simulink model "PLL_Sim_Rev2"  (R2019b)
settings: Solver=VariableStepAuto  StartTime=0.0  StopTime=1  MaxStep=1000  MinStep=1e-10  RelTol=1e-2  AbsTol=1e-2
libraries: fl_lib x17, nesl_utility x8, ee_lib x6, impairlib x2
settings Model: Creator=connerhannon  LastModifiedBy=connerhannon
settings SolverCC: MaxConsecutiveZCs=10000000  MaxConsecutiveMinStep=1000000

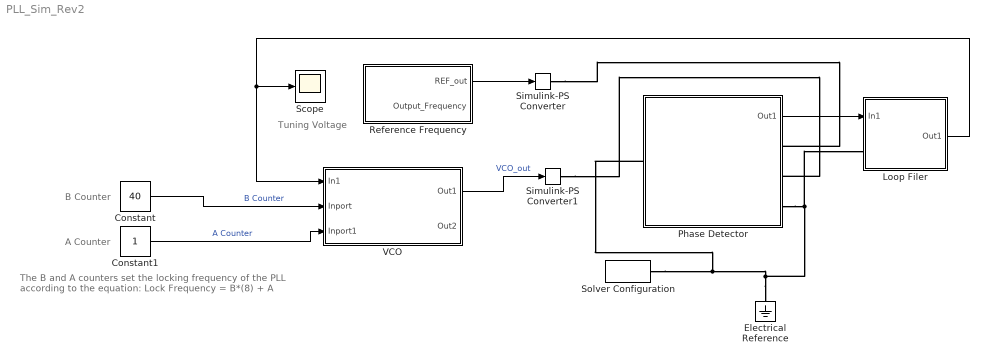
== system PLL_Sim_Rev2 ==
  note: Tuning Voltage
  note: B Counter
  note: The B and A counters set the locking frequency of the PLL
      | according to the equation:
      |
      | Lock Frequency = B*(8) + A
  note: A Counter
  Constant : Constant  Value=40
  Constant1 : Constant
  Electrical Reference : fl_lib/Electrical/Electrical Elements/Electrical Reference
  Loop Filer : Subsystem
  Phase Detector : Subsystem
  Reference Frequency : Subsystem
  Scope : Scope
  Simulink-PS Converter : nesl_utility/Simulink-PS Converter  PhysicalDomain=network_engine_domain  SubClassName=ps_input  LeftPortType=input  RightPortType=output  PseudoPeriodic=off  Frequencies=[]  NoiseDistribution=none  NoiseParameters=[]  Unit=1  AffineConversion=off  FilteringAndDerivatives=provide  SimscapeFilterOrder=1  InputFilterTimeConstant=0.001  UdotUserProvided=0
  Simulink-PS Converter1 : nesl_utility/Simulink-PS Converter  PhysicalDomain=network_engine_domain  SubClassName=ps_input  LeftPortType=input  RightPortType=output  PseudoPeriodic=off  Frequencies=[]  NoiseDistribution=none  NoiseParameters=[]  Unit=1  AffineConversion=off  FilteringAndDerivatives=provide  SimscapeFilterOrder=1  InputFilterTimeConstant=0.001  UdotUserProvided=0
  Solver Configuration : nesl_utility/Solver Configuration  PhysicalDomain=network_engine_domain  SubClassName=solver  LeftPortType=input  RightPortType=generic  Tones=[]  Harmonics=[]  SimulateNoise=off  Profile=off  UseLocalSampling=off  EnableSwitchedLinearOptims=on  FrequencyDomain=off  UseCCode=off  RelTol=0.001  AbsTol=1e-06  MinStep=1e-09  ToWorkspace=off  RevertToSquareIcSolve=off  NumHomotopyIterations=100  PhasorMode=off  PhasorModeNumHarmonics=1  DoDC=off  ResidualTolerance=1e-6  UseLocalSolver=off  LocalSolverChoice=NE_TRAPEZOIDAL_ADVANCER  LocalSolverSampleTime=1e-9  DoFixedCost=off  MaxNonlinIter=3  MaxModeIter=2  LinearAlgebra=auto  EquationFormulation=NE_TIME_EF  DelaysMemoryBudget=1024  AutomaticFiltering=on  FilteringTimeConstant=0.0001  PartitionStorageMethod=AS_NEEDED  PartitionMemoryBudget=1024  PartitionMethod=FAST
  VCO : Subsystem
  wires:
  Constant1/1 -> VCO/3(Inport1)  "A Counter"
  Reference Frequency/1(REF_out) -> Simulink-PS Converter/1
  Constant/1 -> VCO/2(Inport)  "B Counter"
  VCO/1(Out1) -> Simulink-PS Converter1/1  "VCO_out"
  Loop Filer/1(Out1) -> VCO/1(In1), Scope/1
  Phase Detector/1(Out1) -> Loop Filer/1(In1)
  connections:
  Electrical Reference/LConn1 -- Phase Detector/LConn1 -- Solver Configuration/RConn1 -- Phase Detector/RConn3 -- Loop Filer/LConn1
  Simulink-PS Converter/RConn1 -- Phase Detector/RConn1
  Simulink-PS Converter1/RConn1 -- Phase Detector/RConn2

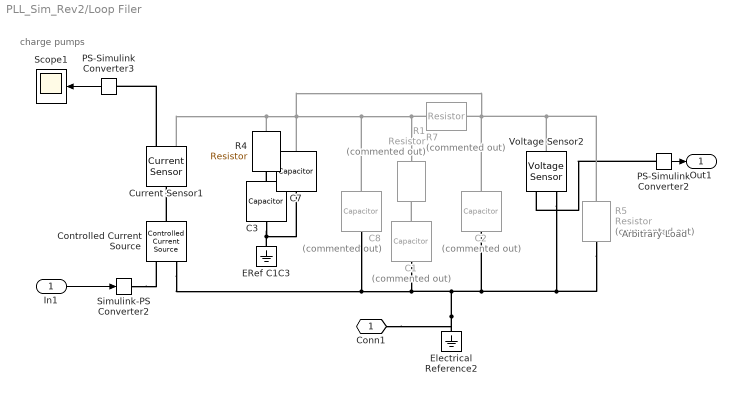
== system PLL_Sim_Rev2/Loop Filer ==
  note: Arbitrary Load
  note: charge pumps
  In1 : Inport
  C1 : fl_lib/Electrical/Electrical Elements/Capacitor  Commented=on  c=80 nF  r=1e-6 Ohm  g=0 1/Ohm  i_specify=off  i_priority=High  i=0 A  i_nominal_specify=off  i_nominal_unit=A  i_nominal_value=1  v_specify=off  v_priority=High  v=0 V  v_nominal_specify=off  v_nominal_unit=V  v_nominal_value=1  vc_specify=on  vc_priority=High  vc=1 V  vc_nominal_specify=off  vc_nominal_unit=V  vc_nominal_value=1
  C2 : fl_lib/Electrical/Electrical Elements/Capacitor  Commented=on  c=220 nF  r=1e-6 Ohm  g=0 1/Ohm  i_specify=off  i_priority=High  i=0 A  i_nominal_specify=off  i_nominal_unit=A  i_nominal_value=1  v_specify=off  v_priority=High  v=0 V  v_nominal_specify=off  v_nominal_unit=V  v_nominal_value=1  vc_specify=on  vc_priority=High  vc=1 V  vc_nominal_specify=off  vc_nominal_unit=V  vc_nominal_value=1
  C3 : fl_lib/Electrical/Electrical Elements/Capacitor  c=82 pF  r=1e-6 Ohm  g=0 1/Ohm  i_specify=off  i_priority=High  i=0 A  i_nominal_specify=off  i_nominal_unit=A  i_nominal_value=1  v_specify=off  v_priority=High  v=0 V  v_nominal_specify=off  v_nominal_unit=V  v_nominal_value=1  vc_specify=on  vc_priority=High  vc=1 V  vc_nominal_specify=off  vc_nominal_unit=V  vc_nominal_value=1
  C7 : fl_lib/Electrical/Electrical Elements/Capacitor  c=17 pF  r=1e-6 Ohm  g=0 1/Ohm  i_specify=off  i_priority=High  i=0 A  i_nominal_specify=off  i_nominal_unit=A  i_nominal_value=1  v_specify=off  v_priority=High  v=0 V  v_nominal_specify=off  v_nominal_unit=V  v_nominal_value=1  vc_specify=on  vc_priority=High  vc=1 V  vc_nominal_specify=off  vc_nominal_unit=V  vc_nominal_value=1
  C8 : fl_lib/Electrical/Electrical Elements/Capacitor  Commented=on  c=12 nF  r=1e-6 Ohm  g=0 1/Ohm  i_specify=off  i_priority=High  i=0 A  i_nominal_specify=off  i_nominal_unit=A  i_nominal_value=1  v_specify=off  v_priority=High  v=0 V  v_nominal_specify=off  v_nominal_unit=V  v_nominal_value=1  vc_specify=on  vc_priority=High  vc=1 V  vc_nominal_specify=off  vc_nominal_unit=V  vc_nominal_value=1
  Controlled Current Source : fl_lib/Electrical/Electrical Sources/Controlled Current Source
  Current Sensor1 : fl_lib/Electrical/Electrical Sensors/Current Sensor
  ERef C1C3 : fl_lib/Electrical/Electrical Elements/Electrical Reference
  Electrical Reference2 : fl_lib/Electrical/Electrical Elements/Electrical Reference
  PS-Simulink Converter2 : nesl_utility/PS-Simulink Converter  PhysicalDomain=network_engine_domain  SubClassName=ps_output  LeftPortType=input  RightPortType=output  PseudoPeriodic=off  Frequencies=[]  Unit=inherit  AffineConversion=off
  PS-Simulink Converter3 : nesl_utility/PS-Simulink Converter  PhysicalDomain=network_engine_domain  SubClassName=ps_output  LeftPortType=input  RightPortType=output  PseudoPeriodic=off  Frequencies=[]  Unit=inherit  AffineConversion=off
  R1 : ee_lib/Passive/Resistor  Commented=on  R=62 kOhm  R_tol=5  enable_R_tol=0  tol_distribution=1  nSigma=4  enable_operating_limits=0  operating_limit_action=2  max_working_voltage=100 V  power_rating=1 W  enable_faults=0  fault_action=1  R_faulted=Inf Ohm  enable_temporal_fault=0  t_fault=1 s  enable_behavioral_fault=0  max_permissible_current=1 A  t_fail_on_current=1 s  noise_mode=0  sample_time=0.001 s  repeatability=1  auto_seed=1646288103  user_seed=0  Tdevice=25 degC  alpha=3.93e-3 1/K  Tmeas=25 degC  thermal_mass=100 J/K  power_derating_T1=70 degC  power_derating_T2=155 degC  operating_temperature_range_vec=[-50, 150] degC  temperature_specify=off  temperature_priority=High  temperature=298.15 K  temperature_nominal_specify=off  temperature_nominal_unit=K  temperature_nominal_value=1
      settings: SourceProductName=Simscape Electrical
  R4 : ee_lib/Passive/Resistor  R=23 kOhm  R_tol=5  enable_R_tol=0  tol_distribution=1  nSigma=4  enable_operating_limits=0  operating_limit_action=2  max_working_voltage=100 V  power_rating=1 W  enable_faults=0  fault_action=1  R_faulted=Inf Ohm  enable_temporal_fault=0  t_fault=1 s  enable_behavioral_fault=0  max_permissible_current=1 A  t_fail_on_current=1 s  noise_mode=0  sample_time=0.001 s  repeatability=1  auto_seed=3563291209  user_seed=0  Tdevice=25 degC  alpha=3.93e-3 1/K  Tmeas=25 degC  thermal_mass=100 J/K  power_derating_T1=70 degC  power_derating_T2=155 degC  operating_temperature_range_vec=[-50, 150] degC  temperature_specify=off  temperature_priority=High  temperature=298.15 K  temperature_nominal_specify=off  temperature_nominal_unit=K  temperature_nominal_value=1
      settings: SourceProductName=Simscape Electrical
  R5 : ee_lib/Passive/Resistor  Commented=on  R=1 kOhm  R_tol=5  enable_R_tol=0  tol_distribution=1  nSigma=4  enable_operating_limits=0  operating_limit_action=2  max_working_voltage=100 V  power_rating=1 W  enable_faults=0  fault_action=1  R_faulted=Inf Ohm  enable_temporal_fault=0  t_fault=1 s  enable_behavioral_fault=0  max_permissible_current=1 A  t_fail_on_current=1 s  noise_mode=0  sample_time=0.001 s  repeatability=1  auto_seed=2651194115  user_seed=0  Tdevice=25 degC  alpha=3.93e-3 1/K  Tmeas=25 degC  thermal_mass=100 J/K  power_derating_T1=70 degC  power_derating_T2=155 degC  operating_temperature_range_vec=[-50, 150] degC  temperature_specify=off  temperature_priority=High  temperature=298.15 K  temperature_nominal_specify=off  temperature_nominal_unit=K  temperature_nominal_value=1
      settings: SourceProductName=Simscape Electrical
  R7 : ee_lib/Passive/Resistor  Commented=on  R=1 kOhm  R_tol=5  enable_R_tol=0  tol_distribution=1  nSigma=4  enable_operating_limits=0  operating_limit_action=2  max_working_voltage=100 V  power_rating=1 W  enable_faults=0  fault_action=1  R_faulted=Inf Ohm  enable_temporal_fault=0  t_fault=1 s  enable_behavioral_fault=0  max_permissible_current=1 A  t_fail_on_current=1 s  noise_mode=0  sample_time=0.001 s  repeatability=1  auto_seed=2471731601  user_seed=0  Tdevice=25 degC  alpha=3.93e-3 1/K  Tmeas=25 degC  thermal_mass=100 J/K  power_derating_T1=70 degC  power_derating_T2=155 degC  operating_temperature_range_vec=[-50, 150] degC  temperature_specify=off  temperature_priority=High  temperature=298.15 K  temperature_nominal_specify=off  temperature_nominal_unit=K  temperature_nominal_value=1
      settings: SourceProductName=Simscape Electrical
  Scope1 : Scope
  Simulink-PS Converter2 : nesl_utility/Simulink-PS Converter  PhysicalDomain=network_engine_domain  SubClassName=ps_input  LeftPortType=input  RightPortType=output  PseudoPeriodic=off  Frequencies=[]  NoiseDistribution=none  NoiseParameters=[]  Unit=1  AffineConversion=off  FilteringAndDerivatives=provide  SimscapeFilterOrder=1  InputFilterTimeConstant=0.001  UdotUserProvided=0
  Voltage Sensor2 : fl_lib/Electrical/Electrical Sensors/Voltage Sensor
  Conn1 : PMIOPort  Side=Left
  Out1 : Outport
  wires:
  PS-Simulink Converter2/1 -> Out1/1
  In1/1 -> Simulink-PS Converter2/1
  PS-Simulink Converter3/1 -> Scope1/1
  connections:
  Simulink-PS Converter2/RConn1 -- Controlled Current Source/RConn1
  Current Sensor1/RConn1 -- PS-Simulink Converter3/LConn1
  PS-Simulink Converter2/LConn1 -- Voltage Sensor2/RConn1
  C1/LConn1 -- R1/RConn1
  Controlled Current Source/LConn1 -- Current Sensor1/LConn1
  R7/LConn1 -- C7/LConn1 -- Current Sensor1/RConn2 -- R4/LConn1 -- C2/LConn1 -- R7/RConn1 -- Voltage Sensor2/LConn1 -- R5/LConn1 -- C8/LConn1 -- R1/LConn1
  Voltage Sensor2/RConn2 -- R5/RConn1 -- Controlled Current Source/RConn2 -- C8/RConn1 -- C1/RConn1 -- Conn1/RConn1 -- Electrical Reference2/LConn1 -- C2/RConn1
  C7/RConn1 -- ERef C1C3/LConn1 -- C3/RConn1
  C3/LConn1 -- R4/RConn1

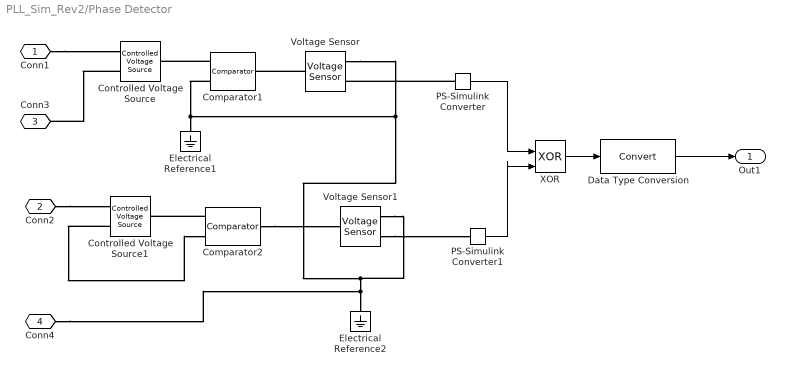
== system PLL_Sim_Rev2/Phase Detector ==
  Comparator1 : ee_lib/Integrated Circuits/Comparator  V_OS=0 mV  V_OL=0 V  V_OH=V_DD V  C_IN=C_iss pF  R_OUT=R Ohm  Delay=t_p s
      settings: SourceProductName=Simscape Electrical  SourceProductBaseCode=PS  InternalSimscapePortConfiguration="{\"Bottom\":[],\"Left\":[{\"id\":\"p\",\"label\":\"+\",\"type\":\"foundation.electrical.electrical\"},{\"id\":\"n\",\"label\":\"-\",\"type\":\"foundation.electrical.electrical\"}],\"Right\":[{\"id\":\"J\",\"label\":\"\",\"type\":\"foundation.electrical.electrical\"}],\"Top\":[]}"
  Comparator2 : ee_lib/Integrated Circuits/Comparator  V_OS=0 mV  V_OL=0 V  V_OH=V_DD V  C_IN=C_iss pF  R_OUT=R Ohm  Delay=t_p s
      settings: SourceProductName=Simscape Electrical  SourceProductBaseCode=PS  InternalSimscapePortConfiguration="{\"Bottom\":[],\"Left\":[{\"id\":\"p\",\"label\":\"+\",\"type\":\"foundation.electrical.electrical\"},{\"id\":\"n\",\"label\":\"-\",\"type\":\"foundation.electrical.electrical\"}],\"Right\":[{\"id\":\"J\",\"label\":\"\",\"type\":\"foundation.electrical.electrical\"}],\"Top\":[]}"
  Controlled Voltage Source : fl_lib/Electrical/Electrical Sources/Controlled Voltage Source
  Controlled Voltage Source1 : fl_lib/Electrical/Electrical Sources/Controlled Voltage Source
  Data Type Conversion : DataTypeConversion
  Electrical Reference1 : fl_lib/Electrical/Electrical Elements/Electrical Reference
  Electrical Reference2 : fl_lib/Electrical/Electrical Elements/Electrical Reference
  PS-Simulink Converter : nesl_utility/PS-Simulink Converter  PhysicalDomain=network_engine_domain  SubClassName=ps_output  LeftPortType=input  RightPortType=output  PseudoPeriodic=off  Frequencies=[]  Unit=inherit  AffineConversion=off
  PS-Simulink Converter1 : nesl_utility/PS-Simulink Converter  PhysicalDomain=network_engine_domain  SubClassName=ps_output  LeftPortType=input  RightPortType=output  PseudoPeriodic=off  Frequencies=[]  Unit=inherit  AffineConversion=off
  Voltage Sensor : fl_lib/Electrical/Electrical Sensors/Voltage Sensor
  Voltage Sensor1 : fl_lib/Electrical/Electrical Sensors/Voltage Sensor
  XOR : Logic  Operator=XOR  IconShape=distinctive  AllPortsSameDT=off  OutDataTypeStr=boolean
  Conn1 : PMIOPort  Side=Right
  Conn2 : PMIOPort  Port=2  Side=Right
  Conn3 : PMIOPort  Port=3  Side=Right
  Conn4 : PMIOPort  Port=4  Side=Left
  Out1 : Outport
  wires:
  Data Type Conversion/1 -> Out1/1
  PS-Simulink Converter/1 -> XOR/1
  PS-Simulink Converter1/1 -> XOR/2
  XOR/1 -> Data Type Conversion/1
  connections:
  Comparator2/RConn1 -- Voltage Sensor1/LConn1
  Voltage Sensor/LConn1 -- Comparator1/RConn1
  Comparator1/LConn2 -- Voltage Sensor1/RConn2 -- Conn4/RConn1 -- Electrical Reference2/LConn1 -- Voltage Sensor/RConn2 -- Electrical Reference1/LConn1
  Comparator1/LConn1 -- Controlled Voltage Source/LConn1
  Conn2/RConn1 -- Controlled Voltage Source1/RConn1
  Controlled Voltage Source1/RConn2 -- Comparator2/LConn2
  Controlled Voltage Source/RConn2 -- Conn3/RConn1
  Conn1/RConn1 -- Controlled Voltage Source/RConn1
  Comparator2/LConn1 -- Controlled Voltage Source1/LConn1
  Voltage Sensor1/RConn1 -- PS-Simulink Converter1/LConn1
  PS-Simulink Converter/LConn1 -- Voltage Sensor/RConn1

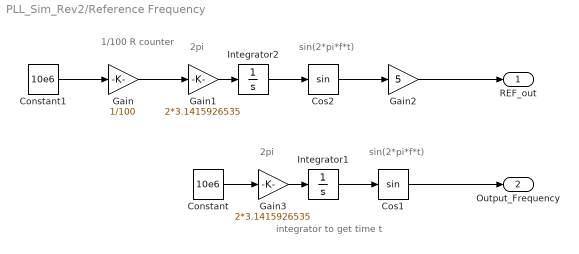
== system PLL_Sim_Rev2/Reference Frequency ==
  note: 1/100
      | R counter
  note: integrator to get time t
  note: sin(2*pi*f*t)
  note: 2pi
  note: sin(2*pi*f*t)
  note: 2pi
  Constant : Constant  Value=10e6
  Constant1 : Constant  Value=10e6
  Cos1 : Trigonometry  OutputSignalType=real
  Cos2 : Trigonometry  OutputSignalType=real
  Gain : Gain  Gain=1/100
  Gain1 : Gain  Gain=2*3.1415926535
  Gain2 : Gain  Gain=5
  Gain3 : Gain  Gain=2*3.1415926535
  Integrator1 : Integrator
  Integrator2 : Integrator
  REF_out : Outport
  "Output_Frequency " : Outport  Port=2
  wires:
  Cos1/1 -> "Output_Frequency "/1
  Gain3/1 -> Integrator1/1
  Integrator1/1 -> Cos1/1
  Constant/1 -> Gain3/1
  Constant1/1 -> Gain/1
  Gain1/1 -> Integrator2/1
  Integrator2/1 -> Cos2/1
  Gain/1 -> Gain1/1
  Cos2/1 -> Gain2/1
  Gain2/1 -> REF_out/1

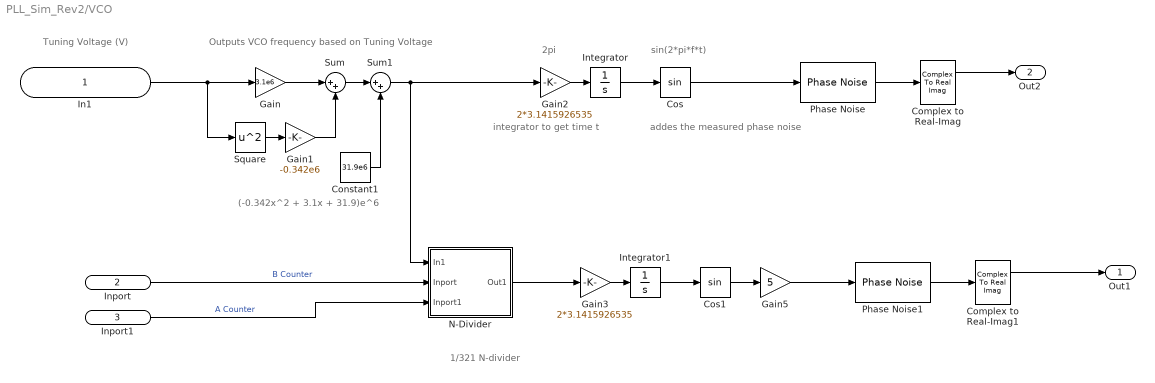
== system PLL_Sim_Rev2/VCO ==
  note: 1/321
      | N-divider
  note: Tuning Voltage
      | (V)
  note: 2pi
  note: sin(2*pi*f*t)
  note: integrator to get time t
  note: (-0.342x^2 + 3.1x + 31.9)e^6
  note: addes the measured phase noise
  note: Outputs VCO frequency based on Tuning Voltage
  In1 : Inport
  Inport : Inport  Port=2
  Inport1 : Inport  Port=3
  Complex to Real-Imag : ComplexToRealImag
  Complex to Real-Imag1 : ComplexToRealImag
  Constant1 : Constant  Value=31.9e6
  Cos : Trigonometry  OutputSignalType=complex
  Cos1 : Trigonometry  OutputSignalType=complex
  Gain : Gain  Gain=3.1e6
  Gain1 : Gain  Gain=-0.342e6
  Gain2 : Gain  Gain=2*3.1415926535
  Gain3 : Gain  Gain=2*3.1415926535
  Gain5 : Gain  Gain=5
  Integrator : Integrator
  Integrator1 : Integrator
  N-Divider : Subsystem
  Phase Noise : impairlib/Phase Noise  Level=[ -36, -73, -83, -90, -112 ]  FrequencyOffset=[ 100, 400, 1000, 5000, 250000]  SampleRate=550000  RandomStream=mt19937ar with seed  Seed=1e6  SimulateUsing=Interpreted execution
      settings: SourceProductName=SerDes Toolbox  SourceProductBaseCode=SX
  Phase Noise1 : impairlib/Phase Noise  Level=[ -36, -73, -83, -90, -112 ]  FrequencyOffset=[ 100, 400, 1000, 5000, 250000]  SampleRate=550000  RandomStream=mt19937ar with seed  Seed=1e6  SimulateUsing=Interpreted execution
      settings: SourceProductName=SerDes Toolbox  SourceProductBaseCode=SX
  Square : Math  Operator=square  SignedPower=off  SaturateOnIntegerOverflow=on
  Sum : Sum  Inputs=|++
  Sum1 : Sum  Inputs=|++
  Out1 : Outport
  Out2 : Outport  Port=2
  wires:
  Gain1/1 -> Sum/2
  Gain/1 -> Sum/1
  Square/1 -> Gain1/1
  Integrator/1 -> Cos/1
  Constant1/1 -> Sum1/2
  Phase Noise/1 -> Complex to Real-Imag/1
  Sum/1 -> Sum1/1
  Cos/1 -> Phase Noise/1
  In1/1 -> Square/1, Gain/1
  Gain2/1 -> Integrator/1
  Gain3/1 -> Integrator1/1
  Phase Noise1/1 -> Complex to Real-Imag1/1
  Cos1/1 -> Gain5/1
  Integrator1/1 -> Cos1/1
  Complex to Real-Imag1/1 -> Out1/1
  Complex to Real-Imag/1 -> Out2/1
  Gain5/1 -> Phase Noise1/1
  Sum1/1 -> N-Divider/1(In1), Gain2/1
  Inport/1 -> N-Divider/2(Inport)  "B Counter"
  Inport1/1 -> N-Divider/3(Inport1)  "A Counter"
  N-Divider/1(Out1) -> Gain3/1

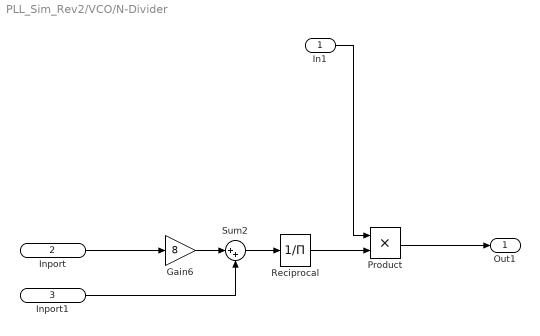
== system PLL_Sim_Rev2/VCO/N-Divider ==
  In1 : Inport
  Inport : Inport  Port=2
  Inport1 : Inport  Port=3
  Gain6 : Gain  Gain=8
  Product : Product
  Reciprocal : Product  Inputs=/
  Sum2 : Sum  Inputs=|++
  Out1 : Outport
  wires:
  Product/1 -> Out1/1
  Inport/1 -> Gain6/1
  Sum2/1 -> Reciprocal/1
  Gain6/1 -> Sum2/1
  Reciprocal/1 -> Product/2
  In1/1 -> Product/1
  Inport1/1 -> Sum2/2
